simulink library "speedgoatlib"  (Simulink 7.3)
settings: Solver=ode45  StartTime=0.0  StopTime=10.0  RelTol=1e-3
undefined symbols (not defined in the file): m_XR17D15x, mmodemcontrol, standard
libraries: speedgoatlib x176, xpclib x88, simulink x4
(part 1 of 4)
Description:
  | 7.14.0.739 (R2012a)
settings Model: sg_rtwmakecfg_data=_sg_IO75X_v1_2_0_  Creator=dkuratli  LastModifiedBy=lab3
settings Model: ForwardingTableString=|
  | ||__slOldName__||speedgoatlib/Utilities/Disable SMIs||__slNewName__||speedgoatlib_utilities/Disable SMIs||__slOldName__||speedgoatlib/IO101/PMC730 1||__slNewName__||speedgoatlib_IO101/Analog input||__slOldName__||speedgoatlib/IO101/PMC730 2||__slNewName__||speedgoatlib_IO101/Analog output||__slOldName__||speedgoatlib/IO101/PMC730 3||__slNewName__||speedgoatlib_IO101/Digital input||__slOldName__||speedgoatlib/IO101/PMC730 4||__slNewName__||speedgoatlib_IO101/Digital output||__slOldName__||speedgoatlib/IO101/PMC730 5||__slNewName__||speedgoatlib_IO101/Setup||__slOldName__||speedgoatlib/IO102/PMC-16AIO 1||__slNewName__||speedgoatlib_IO102/Setup||__slOldName__||speedgoatlib/IO102/PMC-16AIO 2||__slNewName__||speedgoatlib_IO102/Analog input||__slOldName__||speedgoatlib/IO102/PMC-16AIO 3||__slNewName__||speedgoatlib_IO102/Analog output||__slOldName__||speedgoatlib/IO102/PMC-16AIO 4||__slNewName__||speedgoatlib_IO102/Digital input||__slOldName__||speedgoatlib/IO102/PMC-16AIO 5||__slNewName__||speedgoatlib_IO102/Digital output||__slOldName__||speedgoatlib/IO103/PMC-16AIO168 1||__slNewName__||speedgoatlib_IO103/Setup||__slOldName__||speedgoatlib/IO103/PMC-16AIO168 2||__slNewName__||speedgoatlib_IO103/Analog input||__slOldName__||speedgoatlib/IO103/PMC-16AIO168 3||__slNewName__||speedgoatlib_IO103/Analog output||__slOldName__||speedgoatlib/IO103/PMC-16AIO168 4||__slNewName__||speedgoatlib_IO103/Digital output||__slOldName__||speedgoatlib/IO104/PMC66-16AISS8AO4 1||__slNewName__||speedgoatlib_IO104/Setup||__slOldName__||speedgoatlib/IO104/PMC66-16AISS8AO4 2||__slNewName__||speedgoatlib_IO104/Analog input||__slOldName__||speedgoatlib/IO104/PMC66-16AISS8AO4 3||__slNewName__||speedgoatlib_IO104/Analog output||__slOldName__||speedgoatlib/IO104/PMC66-16AISS8AO4 4||__slNewName__||speedgoatlib_IO104/Digital input||__slOldName__||speedgoatlib/IO104/PMC66-16AISS8AO4 5||__slNewName__||speedgoatlib_IO104/Digital output||__slOldName__||speedgoatlib/IO104/PMC66-16AISS8AO4 6||__slNewName__||speedgoatlib_IO104/Start conversion||__slOldName__||speedgoatlib/IO104/PMC66-16AISS8AO4 7||__slNewName__||speedgoatlib_IO104/Read channels||__slOldName__||speedgoatlib/IO104/PMC66-16AISS8AO4 8||__slNewName__||speedgoatlib_IO104/Update channels||__slOldName__||speedgoatlib/IO104/PMC66-16AISS8AO4 9||__slNewName__||speedgoatlib_IO104/Write channels||__slOldName__||speedgoatlib/IO105/PMC-16AI64 1||__slNewName__||speedgoatlib_IO105/Setup||__slOldName__||speedgoatlib/IO105/PMC-16AI64 2||__slNewName__||speedgoatlib_IO105/Analog input||__slOldName__||speedgoatlib/IO106/PMC66-16AI64SSA 1||__slNewName__||speedgoatlib_IO106/Setup||__slOldName__||speedgoatlib/IO106/PMC66-16AI64SSA 2||__slNewName__||speedgoatlib_IO106/Analog input||__slOldName__||speedgoatlib/IO106/PMC66-16AI64SSA 3||__slNewName__||speedgoatlib_IO106/Start conversion||__slOldName__||speedgoatlib/IO106/PMC66-16AI64SSA 4||__slNewName__||speedgoatlib_IO106/Read channels||__slOldName__||speedgoatlib/IO106/PMC66-16AI64SSA 5||__slNewName__||speedgoatlib_IO106/Analog input (DMA)||__slOldName__||speedgoatlib/IO107/PMC66-16AO16 1||__slNewName__||speedgoatlib_IO107/Setup||__slOldName__||speedgoatlib/IO107/PMC66-16AO16 2||__slNewName__||speedgoatlib_IO107/Analog output||__slOldName__||speedgoatlib/IO108/PMC66-16AO16 1||__slNewName__||speedgoatlib_IO108/Setup||__slOldName__||speedgoatlib/IO108/PMC66-16AO16 2||__slNewName__||speedgoatlib_IO108/Analog output||__slOldName__||speedgoatlib/IO110/TPMC553-10 1||__slNewName__||speedgoatlib_IO110/Setup||__slOldName__||speedgoatlib/IO110/TPMC553-10 2||__slNewName__||speedgoatlib_IO110/Analog output||__slOldName__||speedgoatlib/IO111/TPMC553-11 1||__slNewName__||speedgoatlib_IO111/Setup||__slOldName__||speedgoatlib/IO111/TPMC553-11 2||__slNewName__||speedgoatlib_IO111/Analog output||__slOldName__||speedgoatlib/IO112/PMC66-18AI32SSC 1||__slNewName__||speedgoatlib_IO112/Setup||__slOldName__||speedgoatlib/IO112/PMC66-18AI32SSC 2||__slNewName__||speedgoatlib_IO112/Analog input||__slOldName__||speedgoatlib/IO112/PMC66-18AI32SSC 3||__slNewName__||speedgoatlib_IO112/Start conversion||__slOldName__||speedgoatlib/IO112/PMC66-18AI32SSC 4||__slNewName__||speedgoatlib_IO112/Read channels||__slOldName__||speedgoatlib_io113/Setup||__slNewName__||speedgoatlib_IO113/Setup||__slOldName__||speedgoatlib_io113/Analog output||__slNewName__||speedgoatlib_IO113/Analog output||__slOldName__||speedgoatlib_io113/Digital output||__slNewName__||speedgoatlib_IO113/Digital output||__slOldName__||speedgoatlib_io113/Digital input||__slNewName__||speedgoatlib_IO113/Digital input||__slOldName__||speedgoatlib/IO203/TPMC681 1||__slNewName__||speedgoatlib_IO203/Setup||__slOldName__||speedgoatlib/IO203/TPMC681 2||__slNewName__||speedgoatlib_IO203/Read||__slOldName__||speedgoatlib/IO203/TPMC681 3||__slNewName__||speedgoatlib_IO203/Write||__slOldName__||speedgoatlib/IO204/TPMC671 1||__slNewName__||speedgoatlib_IO204/Setup||__slOldName__||speedgoatlib/IO204/TPMC671 2||__slNewName__||speedgoatlib_IO204/Read||__slOldName__||speedgoatlib/IO204/TPMC671 3||__slNewName__||speedgoatlib_IO204/Write||__slOldName__||speedgoatlib/IO205/TPMC700 1||__slNewName__||speedgoatlib_IO205/Setup||__slOldName__||speedgoatlib/IO205/TPMC700 2||__slNewName__||speedgoatlib_IO205/Read||__slOldName__||speedgoatlib/IO205/TPMC700 3||__slNewName__||speedgoatlib_IO205/Write||__slOldName__||speedgoatlib/IO206/TPMC600 1||__slNewName__||speedgoatlib_IO206/Setup||__slOldName__||speedgoatlib/IO206/TPMC600 2||__slNewName__||speedgoatlib_IO206/Read||__slOldName__||speedgoatlib/IO401/TPMC117 1||__slNewName__||speedgoatlib_IO401/Setup||__slOldName__||speedgoatlib/IO401/TPMC117 2||__slNewName__||speedgoatlib_IO401/Incremental encoder||__slOldName__||speedgoatlib/IO401/TPMC117 3||__slNewName__||speedgoatlib_IO401/Absolute SSI encoder||__slOldName__||speedgoatlib/IO401/TPMC117 4||__slNewName__||speedgoatlib_IO401/Simultaneous read||__slOldName__||speedgoatlib/IO503/TPMC466||__slNewName__||speedgoatlib/IO503/Send Receive||__slOldName__||speedgoatlib/IO503/TEWS TPMC466
  | Internal blocks/Setup ||__slNewName__||speedgoatlib/IO503/Speedgoat IO503
  | Internal blocks/Setup||__slOldName__||speedgoatlib/IO503/TEWS TPMC466
  | Internal blocks/Enable TX ||__slNewName__||speedgoatlib/IO503/Speedgoat IO503
  | Internal blocks/Enable TX||__slOldName__||speedgoatlib/IO503/TEWS TPMC466
  | Internal blocks/Read Int Status||__slNewName__||speedgoatlib/IO503/Speedgoat IO503
  | Internal blocks/Read Int Status||__slOldName__||speedgoatlib/IO503/TEWS TPMC466
  | Internal blocks/Board Setup||__slNewName__||speedgoatlib/IO503/Speedgoat IO503
  | Internal blocks/Board Setup||__slOldName__||speedgoatlib/IO503/TEWS TPMC466
  | Internal blocks/Write HW FIFO||__slNewName__||speedgoatlib/IO503/Speedgoat IO503
  | Internal blocks/Write HW FIFO||__slOldName__||speedgoatlib/IO503/TEWS TPMC466
  | Internal blocks/Read HW FIFO||__slNewName__||speedgoatlib/IO503/Speedgoat IO503
  | Internal blocks/Read HW FIFO||__slOldName__||speedgoatlib/IO503/TEWS TPMC466
  | Internal blocks/Int Source Filter||__slNewName__||speedgoatlib/IO503/Speedgoat IO503
  | Internal blocks/Int Source Filter||__slOldName__||speedgoatlib/IO504/TPMC465||__slNewName__||speedgoatlib/IO504/Send Receive||__slOldName__||speedgoatlib/IO504/TEWS TPMC465
  | Internal blocks/Setup ||__slNewName__||speedgoatlib/IO504/Speedgoat IO504
  | Internal blocks/Setup||__slOldName__||speedgoatlib/IO504/TEWS TPMC465
  | Internal blocks/Read Int Status||__slNewName__||speedgoatlib/IO504/Speedgoat IO504
  | Internal blocks/Read Int Status||__slOldName__||speedgoatlib/IO504/TEWS TPMC465
  | Internal blocks/Board Setup||__slNewName__||speedgoatlib/IO504/Speedgoat IO504
  | Internal blocks/Board Setup||__slOldName__||speedgoatlib/IO504/TEWS TPMC465
  | Internal blocks/Enable TX ||__slNewName__||speedgoatlib/IO504/Speedgoat IO504 Internal blocks/Enable TX||__slOldName__||speedgoatlib/IO504/TEWS TPMC465
  | Internal blocks/Write HW FIFO||__slNewName__||speedgoatlib/IO504/Speedgoat IO504
  | Internal blocks/Write HW FIFO||__slOldName__||speedgoatlib/IO504/TEWS TPMC465
  | Internal blocks/Read HW FIFO||__slNewName__||speedgoatlib/IO504/Speedgoat IO504
  | Internal blocks/Read HW FIFO||__slOldName__||speedgoatlib/IO504/TEWS TPMC465
  | Internal blocks/Int Source Filter||__slNewName__||speedgoatlib/IO504/Speedgoat IO504
  | Internal blocks/Int Source Filter||__slOldName__||speedgoatlib/IO601/iPC-I XC16//PMC 1||__slNewName__||speedgoatlib_IO601/Setup||__slOldName__||speedgoatlib/IO601/iPC-I XC16//PMC 2||__slNewName__||speedgoatlib_IO601/Obsolete/Write||__slOldName__||speedgoatlib/IO601/iPC-I XC16//PMC 3||__slNewName__||speedgoatlib_IO601/Obsolete Read||__slOldName__||speedgoatlib/IO601/iPC-I XC16//PMC 4||__slNewName__||speedgoatlib_IO601/Combined read||__slOldName__||speedgoatlib/IO601/iPC-I XC16//PMC 5||__slNewName__||speedgoatlib_IO601/Status||__slOldName__||speedgoatlib/IO601/iPC-I XC16//PMC 6||__slNewName__||speedgoatlib_IO601/Read status||__slOldName__||speedgoatlib/IO601/iPC-I XC16//PMC 7||__slNewName__||speedgoatlib_IO601/Read status CAN port||__slOldName__||speedgoatlib/IO601/iPC-I XC16//PMC 8||__slNewName__||speedgoatlib_IO601/Send||__slOldName__||speedgoatlib/IO601/iPC-I XC16//PMC 9||__slNewName__||speedgoatlib_IO601/Receive||__slOldName__||speedgoatlib/IO601/iPC-I XC16//PMC 12 v2||__slNewName__||speedgoatlib_IO601/Write||__slOldName__||speedgoatlib/IO601/iPC-I XC16//PMC 13 v2||__slNewName__||speedgoatlib_IO601/Read

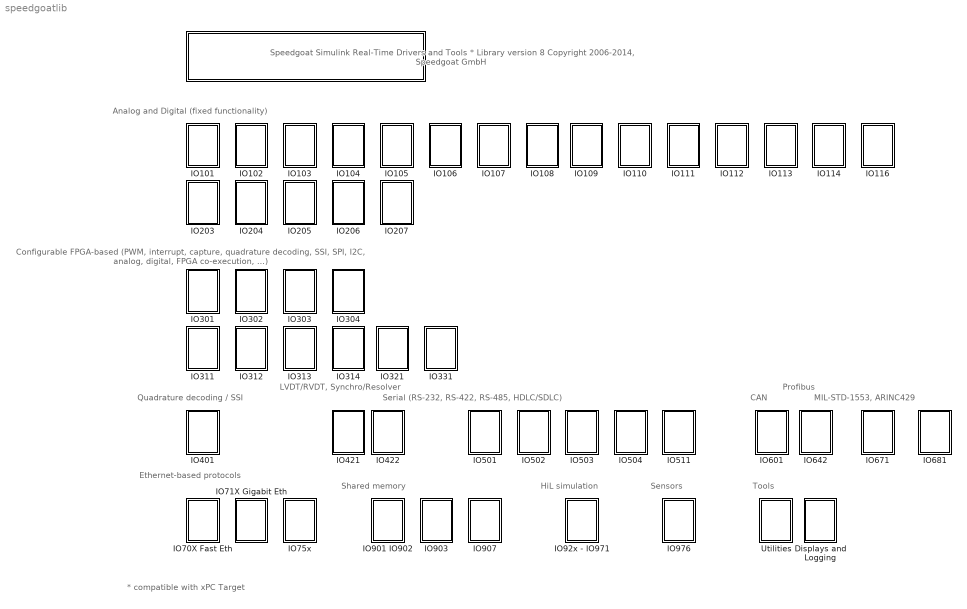
== system speedgoatlib ==
  note: * compatible with xPC Target
  note: Speedgoat Simulink Real-Time Drivers and Tools *
      | Library version 8
      | Copyright 2006-2014, Speedgoat GmbH
  note: Analog and Digital (fixed functionality)
  note: Configurable FPGA-based (PWM, interrupt, capture, quadrature decoding, SSI, SPI, I2C, analog, digital, FPGA co-execution, ...)
  note: Quadrature decoding / SSI
  note: Serial (RS-232, RS-422, RS-485, HDLC/SDLC)
  note: CAN
  note: Ethernet-based protocols
  note: Shared memory
  note: Tools
  note: HiL simulation
  note: Sensors
  note: MIL-STD-1553, ARINC429
  note: LVDT/RVDT, Synchro/Resolver
  note: Profibus
  " " : Subsystem
      settings: OpenFcn=;
      mask Display: image(imread('sg_logo.png'))
  Displays and Logging : Subsystem
      settings: OpenFcn=|
      | [matlabVer, count] = sscanf(version, '%i.%i.%i');
      | 
      | if (matlabVer(1) < 7) || ( (matlabVer(1) == 8) && (matlabVer(2) <= 2) )
      |   load_system('xpclib');
      |   open_system('xpclib/Misc.');
      | else
      |   load_system('slrtlib');
      |   open_system('slrtlib/Displays and Logging');
      | end
  IO101 : Subsystem
      settings: OpenFcn=speedgoatlib_IO101
  IO102 : Subsystem
      settings: OpenFcn=speedgoatlib_IO102
  IO103 : Subsystem
      settings: OpenFcn=speedgoatlib_IO103
  IO104 : Subsystem
      settings: OpenFcn=speedgoatlib_IO104
  IO105 : Subsystem
      settings: OpenFcn=speedgoatlib_IO105
  IO106 : Subsystem
      settings: OpenFcn=speedgoatlib_IO106
  IO107 : Subsystem
      settings: OpenFcn=speedgoatlib_IO107
  IO108 : Subsystem
      settings: OpenFcn=speedgoatlib_IO108
  IO109 : Subsystem
      settings: OpenFcn=speedgoatlib_IO109
  IO110 : Subsystem
      settings: OpenFcn=speedgoatlib_IO110
  IO111 : Subsystem
      settings: OpenFcn=speedgoatlib_IO111
  IO112 : Subsystem
      settings: OpenFcn=speedgoatlib_IO112
  IO113 : Subsystem
      settings: OpenFcn=speedgoatlib_IO113
  IO114 : Subsystem
      settings: OpenFcn=speedgoatlib_IO114
  IO116 : Subsystem
      settings: OpenFcn=speedgoatlib_IO116
  IO203 : Subsystem
      settings: OpenFcn=speedgoatlib_IO203
  IO204 : Subsystem
      settings: OpenFcn=speedgoatlib_IO204
  IO205 : Subsystem
      settings: OpenFcn=speedgoatlib_IO205
  IO206 : Subsystem
      settings: OpenFcn=speedgoatlib_IO206
  IO207 : Subsystem
      settings: OpenFcn=speedgoatlib_IO207
  IO301 : Subsystem
      settings: OpenFcn=speedgoatlib_IO301
  IO302 : Subsystem
      settings: OpenFcn=speedgoatlib_IO302
  IO303 : Subsystem
      settings: OpenFcn=speedgoatlib_IO303
  IO304 : Subsystem
      settings: OpenFcn=speedgoatlib_IO304
  IO311 : Subsystem
      settings: OpenFcn=speedgoatlib_IO311
  IO312 : Subsystem
      settings: OpenFcn=speedgoatlib_IO312
  IO313 : Subsystem
      settings: OpenFcn=speedgoatlib_IO313
  IO314 : Subsystem
      settings: OpenFcn=speedgoatlib_IO314
  IO321 : Subsystem
      settings: OpenFcn=speedgoatlib_IO321
  IO331 : Subsystem
      settings: OpenFcn=speedgoatlib_fpga
  IO401 : Subsystem
      settings: OpenFcn=speedgoatlib_IO401
  IO421 : Subsystem
      settings: OpenFcn=speedgoatlib_IO421
  IO422 : Subsystem
      settings: OpenFcn=speedgoatlib_IO422
  IO501 : Subsystem
  IO502 : Subsystem
  IO503 : Subsystem
  IO504 : Subsystem
  IO511 : Subsystem
      settings: OpenFcn=speedgoatlib_IO511
  IO601 : Subsystem
      settings: OpenFcn=speedgoatlib_IO601
  IO642 : Subsystem
      settings: OpenFcn=speedgoatlib_IO642
  IO671 : Subsystem
      settings: OpenFcn=|
      | load_system('xpccondorlib');
      | open_system('xpccondorlib/MIL-STD 1553');
  IO681 : Subsystem
      settings: OpenFcn=|
      | load_system('xpccondorlib');
      | open_system('xpccondorlib/ARINC-429');
  IO70X Fast Eth : Subsystem
      settings: OpenFcn=speedgoatlib_IO70X
  IO71X Gigabit Eth : Subsystem
      settings: OpenFcn=speedgoatlib_IO71X
  IO75x : Subsystem
      settings: OpenFcn=speedgoatlib_IO75X
  IO901 IO902 : Subsystem
      settings: OpenFcn=cwcec_scgtLib
  IO903 : Subsystem
      settings: OpenFcn=|
      | open_system('xpcsystranlib');
      | open_system('xpcsystranlib/Shared Memory');
  IO907 : Subsystem
      settings: OpenFcn=|
      | load_system('xpcgefanuclib');
      | open_system('xpcgefanuclib/Shared Memory');
  IO92x - IO971 : Subsystem
      settings: OpenFcn=speedgoatlib_PIL
  IO976 : Subsystem
      settings: OpenFcn=|
      | load_system('xpcmeasurementcomputinglib');
      | open_system('xpcmeasurementcomputinglib/Thermo couple');
  Utilities : Subsystem
      settings: OpenFcn=speedgoatlib_utilities

== system speedgoatlib/  ==

== system speedgoatlib/Displays and Logging ==

== system speedgoatlib/IO101 ==

== system speedgoatlib/IO102 ==

== system speedgoatlib/IO103 ==

== system speedgoatlib/IO104 ==

== system speedgoatlib/IO105 ==

== system speedgoatlib/IO106 ==

== system speedgoatlib/IO107 ==

== system speedgoatlib/IO108 ==

== system speedgoatlib/IO109 ==

== system speedgoatlib/IO110 ==

== system speedgoatlib/IO111 ==

== system speedgoatlib/IO112 ==

== system speedgoatlib/IO113 ==

== system speedgoatlib/IO114 ==

== system speedgoatlib/IO116 ==

== system speedgoatlib/IO203 ==

== system speedgoatlib/IO204 ==

== system speedgoatlib/IO205 ==

== system speedgoatlib/IO206 ==

== system speedgoatlib/IO207 ==

== system speedgoatlib/IO301 ==

== system speedgoatlib/IO302 ==

== system speedgoatlib/IO303 ==

== system speedgoatlib/IO304 ==

== system speedgoatlib/IO311 ==

== system speedgoatlib/IO312 ==

== system speedgoatlib/IO313 ==

== system speedgoatlib/IO314 ==

== system speedgoatlib/IO321 ==

== system speedgoatlib/IO331 ==

== system speedgoatlib/IO401 ==

== system speedgoatlib/IO421 ==

== system speedgoatlib/IO422 ==

== system speedgoatlib/IO501 ==
  Acromag PMC520 Internal blocks : Subsystem
  Modem Control : S-Function  InitFcn=mmodemcontrol(3)  FunctionName=modem_control_XR17D15x  Parameters=slot, port, boardtype, rts, dtr, count  EnableBusSupport=off  mask(modem_control_XR17D15x){port=1, rts=on, dtr=off, slot=[2,13]}
      mask prompts: slot "PCI slot: (-1 for autosearch)"
      mask help:
      | PMC520
      | Acromag
      | Modem Control
      mask init:
      | count = 0;
      | boardtype = 100;
      | [maskdisplay, count] = mmodemcontrol( 2, rts, dtr, boardtype, 0, 0 );
      | set_param( gcb, 'MaskDisplay', maskdisplay );
      mask Help: helpview(fullfile(docroot, 'mapfiles', 'xpc.map'), 'Quatech_MODEM_Control')
      mask StyleString: popup(1|2),checkbox,checkbox,edit
      mask Display: disp('PMC520\nAcromag\nModem Control');port_label('input',1,'RTS');
  Modem Status : S-Function  FunctionName=modem_status_XR17D15x  Parameters=slot, port, boardtype, cts, dsr, ring, dcd, count, sampletime  EnableBusSupport=off  mask(modem_status_XR17D15x){port=1, cts=on, dsr=off, ring=off, dcd=off, sampletime=-1, slot=[2,13]}
      mask prompts: ring "RI:"; slot "PCI slot: (-1 for autosearch)"
      mask help:
      | PMC520
      | Acromag
      | Modem Status
      mask init:
      | count = 0;
      | boardtype = 100;
      | [maskdisplay, count] = mmodemstatus( 2, cts, dsr, ring, dcd, boardtype );
      | set_param( gcb, 'MaskDisplay', maskdisplay );
      mask Help: helpview(fullfile(docroot, 'mapfiles', 'xpc.map'), 'FC422_MODEM_Status')
      mask StyleString: popup(1|2),checkbox,checkbox,checkbox,checkbox,edit,edit
      mask Display: disp('PMC520\nAcromag\nModem Control');port_label('output',1,'CTS');
  PMC520 : Subsystem  InitFcn=m_XR17D15x(3);  mask(RS232 Send Receive){group=Board Setup, port=1, irqnum=5, clockfreq=14745600, standard=on, slot=-1, baud1=115200, bauddivisor1=1, sampling1=16x (standard), prescale1=off, parity1=None, ndata1=8, nstop1=1, rlevel1=1, hwmode1=none, swmode1=none, xonchar1=17, xoffchar1=19, rs485auto1=off, rs485delay1=0, xmtfifosize1=1024, xmtdatatype1=8 bit uint null terminated, rcvfifosize1=1024, baud2=115200, bauddivisor2=1, sampling2=16x (standard), prescale2=off, parity2=None, ndata2=8, nstop2=1, rlevel2=1, hwmode2=none, swmode2=none, xonchar2=17, xoffchar2=19, rs485auto2=off, rs485delay2=0, xmtfifosize2=1024, xmtdatatype2=8 bit uint null terminated, rcvfifosize2=1024, baud3=115200, bauddivisor3=1, sampling3=16x (standard), prescale3=off, parity3=None, ndata3=8, nstop3=1, rlevel3=half full (32), hwmode3=none, swmode3=none, xonchar3=17, xoffchar3=19, rs485auto3=off, rs485delay3=0, xmtfifosize3=1024, xmtdatatype3=8 bit uint null terminated, rcvfifosize3=1024, baud4=115200, bauddivisor4=1, sampling4=16x (standard), prescale4=off, parity4=None, ndata4=8, nstop4=1, rlevel4=half full (32), hwmode4=none, swmode4=none, xonchar4=17, xoffchar4=19, rs485auto4=off, rs485delay4=0, xmtfifosize4=1024, xmtdatatype4=8 bit uint null terminated, rcvfifosize4=1024, baud5=115200, bauddivisor5=1, sampling5=16x (standard), prescale5=off, parity5=None, ndata5=8, nstop5=1, rlevel5=1, hwmode5=none, swmode5=none, xonchar5=17, xoffchar5=19, rs485auto5=off, rs485delay5=0, xmtfifosize5=1024, xmtdatatype5=8 bit uint null terminated, rcvfifosize5=1024, baud6=115200, bauddivisor6=1, sampling6=16x (standard), prescale6=off, parity6=None, ndata6=8, nstop6=1, rlevel6=1, hwmode6=none, swmode6=none, xonchar6=17, xoffchar6=19, rs485auto6=off, rs485delay6=0, xmtfifosize6=1024, xmtdatatype6=8 bit uint null terminated, rcvfifosize6=1024, baud7=115200, bauddivisor7=1, sampling7=16x (standard), prescale7=off, parity7=None, ndata7=8, nstop7=1, rlevel7=1, hwmode7=none, swmode7=none, xonchar7=17, xoffchar7=19, rs485auto7=off, rs485delay7=0, xmtfifosize7=1024, xmtdatatype7=8 bit uint null terminated, rcvfifosize7=1024, baud8=115200, bauddivisor8=1, sampling8=16x (standard), prescale8=off, parity8=None, ndata8=8, nstop8=1, rlevel8=1, hwmode8=none, swmode8=none, xonchar8=17, xoffchar8=19, rs485auto8=off, rs485delay8=0, xmtfifosize8=1024, xmtdatatype8=8 bit uint null terminated, rcvfifosize8=1024}
      mask prompts: group "Parameter group:"; port "Port to modify:"; irqnum "IRQ number:"; clockfreq "Master Clock Frequeny (standard = 14.7456E6 Hz):"; standard "Use standard reference and rates (Ref = 14.7456E6 Hz, 16x sampling, all ports)"; baud1 "Baud rate:"; bauddivisor1 "Baud divisor:"; sampling1 "Sampling rate:"; prescale1 "Prescale (divide reference by 4)"; parity1 "Parity:"; ndata1 "Data bits:"; nstop1 "Stop bits:"; rlevel1 "Receive FIFO interrupt level:"; hwmode1 "Hardware handshake:"; swmode1 "Software handshake:"; xonchar1 "XON character:"; xoffchar1 "XOFF character:"; rs485auto1 "RS485 auto turnaround:"; rs485delay1 "RS485 turnaround delay [0,15]"; xmtfifosize1 "Transmit software FIFO size:"; xmtdatatype1 "Transmit FIFO data type:"; rcvfifosize1 "Receive software FIFO size:"; baud2 "Baud rate:"; bauddivisor2 "Baud divisor:"; sampling2 "Sampling rate:"; prescale2 "Prescale (divide reference by 4)"; parity2 "Parity:"; ndata2 "Data bits:"; nstop2 "Stop bits:"; rlevel2 "Receive FIFO interrupt level:"; hwmode2 "Hardware handshake:"; swmode2 "Software handshake:"; xonchar2 "XON character:"; xoffchar2 "XOFF character:"; rs485auto2 "RS485 auto turnaround:"; rs485delay2 "RS485 turnaround delay [0,15]"; xmtfifosize2 "Transmit software FIFO size:"; xmtdatatype2 "Transmit FIFO data type:"; rcvfifosize2 "Receive software FIFO size:"; baud3 "Baud rate:"; bauddivisor3 "Baud divisor:"; sampling3 "Sampling rate:"; prescale3 "Prescale (divide reference by 4)"; parity3 "Parity:"; ndata3 "Data bits:"; nstop3 "Stop bits:"; rlevel3 "Receive FIFO interrupt level:"; hwmode3 "Hardware handshake:"; swmode3 "Software handshake:"; xonchar3 "XON character:"; xoffchar3 "XOFF character:"; rs485auto3 "RS485 auto turnaround:"; rs485delay3 "RS485 turnaround delay [0,15]"; xmtfifosize3 "Transmit software FIFO size:"; xmtdatatype3 "Transmit FIFO data type:"; rcvfifosize3 "Receive software FIFO size:"; baud4 "Baud rate:"; bauddivisor4 "Baud divisor:"; sampling4 "Sampling rate:"; prescale4 "Prescale (divide reference by 4)"; parity4 "Parity:"; ndata4 "Data bits:"; nstop4 "Stop bits:"; rlevel4 "Receive FIFO interrupt level:"; hwmode4 "Hardware handshake:"; swmode4 "Software handshake:"; xonchar4 "XON character:"; xoffchar4 "XOFF character:"; rs485auto4 "RS485 auto turnaround:"; rs485delay4 "RS485 turnaround delay [0,15]"; xmtfifosize4 "Transmit software FIFO size:"; xmtdatatype4 "Transmit FIFO data type:"; rcvfifosize4 "Receive software FIFO size:"; baud5 "Baud rate:"; bauddivisor5 "Baud divisor:"; sampling5 "Sampling rate:"; prescale5 "Prescale (divide reference by 4)"; parity5 "Parity:"; ndata5 "Data bits:"; nstop5 "Stop bits:"; rlevel5 "Receive FIFO interrupt level:"; hwmode5 "Hardware handshake:"; swmode5 "Software handshake:"; xonchar5 "XON character:"; xoffchar5 "XOFF character:"; rs485auto5 "RS485 auto turnaround:"; rs485delay5 "RS485 turnaround delay [0,15]"; xmtfifosize5 "Transmit software FIFO size:"; xmtdatatype5 "Transmit FIFO data type:"; rcvfifosize5 "Receive software FIFO size:"; baud6 "Baud rate:"; bauddivisor6 "Baud divisor:"; sampling6 "Sampling rate:"; prescale6 "Prescale (divide reference by 4)"; parity6 "Parity:"; ndata6 "Data bits:"; nstop6 "Stop bits:"; rlevel6 "Receive FIFO interrupt level:"; hwmode6 "Hardware handshake:"; swmode6 "Software handshake:"; xonchar6 "XON character:"; xoffchar6 "XOFF character:"; rs485auto6 "RS485 auto turnaround:"; rs485delay6 "RS485 turnaround delay [0,15]"; xmtfifosize6 "Transmit software FIFO size:"; xmtdatatype6 "Transmit FIFO data type:"; rcvfifosize6 "Receive software FIFO size:"; baud7 "Baud rate:"; bauddivisor7 "Baud divisor:"; sampling7 "Sampling rate:"; prescale7 "Prescale (divide reference by 4)"; parity7 "Parity:"; ndata7 "Data bits:"; nstop7 "Stop bits:"; rlevel7 "Receive FIFO interrupt level:"; hwmode7 "Hardware handshake:"; swmode7 "Software handshake:"; xonchar7 "XON character:"; xoffchar7 "XOFF character:"; rs485auto7 "RS485 auto turnaround:"; rs485delay7 "RS485 turnaround delay [0,15]"; xmtfifosize7 "Transmit software FIFO size:"; xmtdatatype7 "Transmit FIFO data type:"; rcvfifosize7 "Receive software FIFO size:"; baud8 "Baud rate:"; bauddivisor8 "Baud divisor:"; sampling8 "Sampling rate:"; prescale8 "Prescale (divide reference by 4)"; parity8 "Parity:"; ndata8 "Data bits:"; nstop8 "Stop bits:"; rlevel8 "Receive FIFO interrupt level:"; hwmode8 "Hardware handshake:"; swmode8 "Software handshake:"; xonchar8 "XON character:"; xoffchar8 "XOFF character:"; rs485auto8 "RS485 auto turnaround:"; rs485delay8 "RS485 turnaround delay [0,15]"; xmtfifosize8 "Transmit software FIFO size:"; xmtdatatype8 "Transmit FIFO data type:"; rcvfifosize8 "Receive software FIFO size:"
      mask help:
      | PMC520
      | Acromag
      | RS232 Send Receive Subsystem
      mask init:
      | brdslot = slot;
      | m_XR17D15x(1, 8);
      mask Help: helpview(fullfile(docroot, 'mapfiles', 'xpc.map'), 'Commtech_Subsystem')
      mask StyleString: popup(Board Setup|Basic Setup|FIFO Setup),popup(1|2|3|4|5|6|7|8),edit,edit,checkbox,edit,popup(921600|460800|230400|115200|57600|38400|19200|9600|4800|2400|1200|600|300|110),edit,popup(8x|16x (standard)),checkbox,popup(None|Even|Odd|Mark|Space),popup(5|6|7|8),popup(1|2),popup(1|quarter full (16)|half full (32)|almost full (56)),popup(RTS/CTS|none),popup(XON/XOFF|none),edit,edit,checkbox,edit,edit,popup(count+32 bit int|count+32 bit uint|count+16 bit int|count+16 bit uint|8 bit int null terminated|8 bit uint null terminated),edit,popup(921600|460800|230400|115200|57600|38400|19200|9600|4800|2400|1200|600|300|110),edit,popup(8x|16x (standard)),checkbox,popup(None|Even|Odd|Mark|Space),popup(5|6|7|8),popup(1|2),popup(1|quarter full (16)|half full (32)|almost full (56)),popup(RTS/CTS|none),popup(XON/XOFF|none),edit,edit,checkbox,edit,edit,popup(count+32 bit int|count+32 bit uint|count+16 bit int|count+16 bit uint|8 bit int null terminated|8 bit uint null terminated),edit,popup(921600|460800|230400|115200|57600|38400|19200|9600|4800|2400|1200|600|300|110),edit,popup(8x|16x (standard)),checkbox,popup(None|Even|Odd|Mark|Space),popup(5|6|7|8),popup(1|2),popup(1|quarter full (16)|half full (32)|almost full (56)),popup(RTS/CTS|none),popup(XON/XOFF|none),edit,edit,checkbox,edit,edit,popup(count+32 bit int|count+32 bit uint|count+16 bit int|count+16 bit uint|8 bit int null terminated|8 bit uint null terminated),edit,popup(921600|460800|230400|115200|57600|38400|19200|9600|4800|2400|1200|600|300|110),edit,popup(8x|16x (standard)),checkbox,popup(None|Even|Odd|Mark|Space),popup(5|6|7|8),popup(1|2),popup(1|quarter full (16)|half full (32)|almost full (56)),popup(RTS/CTS|none),popup(XON/XOFF|none),edit,edit,checkbox,edit,edit,popup(count+32 bit int|count+32 bit uint|count+16 bit int|count+16 bit uint|8 bit int null terminated|8 bit uint null terminated),edit,popup(921600|460800|230400|115200|57600|38400|19200|9600|4800|2400|1200|600|300|110),edit,popup(8x|16x (standard)),checkbox,popup(None|Even|Odd|Mark|Space),popup(5|6|7|8),popup(1|2),popup(1|quarter full (16)|half full (32)|almost full (56)),popup(RTS/CTS|none),popup(XON/XOFF|none),edit,edit,checkbox,edit,edit,popup(count+32 bit int|count+32 bit uint|count+16 bit int|count+16 bit uint|8 bit int null terminated|8 bit uint null terminated),edit,popup(921600|460800|230400|115200|57600|38400|19200|9600|4800|2400|1200|600|300|110),edit,popup(8x|16x (standard)),checkbox,popup(None|Even|Odd|Mark|Space),popup(5|6|7|8),popup(1|2),popup(1|quarter full (16)|half full (32)|almost full (56)),popup(RTS/CTS|none),popup(XON/XOFF|none),edit,edit,checkbox,edit,edit,popup(count+32 bit int|count+32 bit uint|count+16 bit int|count+16 bit uint|8 bit int null terminated|8 bit uint null terminated),edit,popup(921600|460800|230400|115200|57600|38400|19200|9600|4800|2400|1200|600|300|110),edit,popup(8x|16x (standard)),checkbox,popup(None|Even|Odd|Mark|Space),popup(5|6|7|8),popup(1|2),popup(1|quarter full (16)|half full (32)|almost full (56)),popup(RTS/CTS|none),popup(XON/XOFF|none),edit,edit,checkbox,edit,edit,popup(count+32 bit int|count+32 bit uint|count+16 bit int|count+16 bit uint|8 bit int null terminated|8 bit uint null terminated),edit,popup(921600|460800|230400|115200|57600|38400|19200|9600|4800|2400|1200|600|300|110),edit,popup(8x|16x (standard)),checkbox,popup(None|Even|Odd|Mark|Space),popup(5|6|7|8),popup(1|2),popup(1|quarter full (16)|half full (32)|almost full (56)),popup(RTS/CTS|none),popup(XON/XOFF|none),edit,edit,checkbox,edit,edit,popup(count+32 bit int|count+32 bit uint|count+16 bit int|count+16 bit uint|8 bit int null terminated|8 bit uint null terminated),edit
      mask CallbackString:
      | m_XR17D15x(2, 8);|m_XR17D15x(2, 8);|||m_XR17D15x(2, 8);
      | |||||||||||||||||||||||||||||||||||||||||||||||||||||||||||||||||||||||||||||||||||||||||||||||||||||||||||||||||||||||||||||||||||||||||
      mask Display:
      | disp('Acromag\nPMC520\nRS-232\nSend\nReceive');
      | port_label( 'input', 1, 'XMT1' );
      | port_label( 'input', 2, 'XMT2' );
      | port_label( 'input', 3, 'XMT3' );
      | port_label( 'input', 4, 'XMT4' );
      | port_label( 'input', 5, 'XMT5' );
      | port_label( 'input', 6, 'XMT6' );
      | port_label( 'input', 7, 'XMT7' );
      | port_label( 'input', 8, 'XMT8' );
      | 
      | port_label( 'output', 1, 'FIFO1' );
      | port_label( 'output', 2, 'FIFO2' );
      | port_label( 'output', 3, 'FIFO3' );
      | port_label( 'output', 4, 'FIFO4' );
      | port_label( 'output', 5, 'FIFO5' );
      | port_label( 'output', 6, 'FIFO6' );
      | port_label( 'output', 7, 'FIFO7' );
      | port_label( 'output', 8, 'FIFO8' );

== system speedgoatlib/IO502 ==
  Acromag PMC521 Internal blocks : Subsystem
  Modem Control : S-Function  InitFcn=mmodemcontrol(3)  FunctionName=modem_control_XR17D15x  Parameters=slot, port, boardtype, rts, dtr, count  EnableBusSupport=off  mask(modem_control_XR17D15x){port=1, rts=on, dtr=off, slot=[2,13]}
      mask prompts: slot "PCI slot: (-1 for autosearch)"
      mask help:
      | PMC521
      | Acromag
      | Modem Control
      mask init:
      | count = 0;
      | boardtype = 101;
      | [maskdisplay, count] = mmodemcontrol( 2, rts, dtr, boardtype, 0, 0 );
      | set_param( gcb, 'MaskDisplay', maskdisplay );
      mask Help: helpview(fullfile(docroot, 'mapfiles', 'xpc.map'), 'Quatech_MODEM_Control')
      mask StyleString: popup(1|2),checkbox,checkbox,edit
      mask Display: disp('Speedgoat\nIO502\nModem Control');port_label('input',1,'RTS');
  Modem Status : S-Function  FunctionName=modem_status_XR17D15x  Parameters=slot, port, boardtype, cts, dsr, ring, dcd, count, sampletime  EnableBusSupport=off  mask(modem_status_XR17D15x){port=1, cts=on, dsr=off, ring=off, dcd=off, sampletime=-1, slot=[2,13]}
      mask prompts: ring "RI:"; slot "PCI slot: (-1 for autosearch)"
      mask help:
      | PMC521
      | Acromag
      | Modem Status
      mask init:
      | count = 0;
      | boardtype = 101;
      | [maskdisplay, count] = mmodemstatus( 2, cts, dsr, ring, dcd, boardtype );
      | set_param( gcb, 'MaskDisplay', maskdisplay );
      mask Help: helpview(fullfile(docroot, 'mapfiles', 'xpc.map'), 'FC422_MODEM_Status')
      mask StyleString: popup(1|2),checkbox,checkbox,checkbox,checkbox,edit,edit
      mask Display: disp('Speedgoat\nIO502\nModem Status');port_label('output',1,'CTS');
  PMC521 : Subsystem  InitFcn=m_XR17D15x(3);  mask(RS232 Send Receive){group=Board Setup, port=1, irqnum=5, clockfreq=14745600, standard=on, slot=-1, baud1=115200, bauddivisor1=1, sampling1=16x (standard), prescale1=off, parity1=None, ndata1=8, nstop1=1, rlevel1=1, hwmode1=none, swmode1=none, xonchar1=17, xoffchar1=19, rs485auto1=off, rs485delay1=0, xmtfifosize1=1024, xmtdatatype1=8 bit uint null terminated, rcvfifosize1=1024, baud2=115200, bauddivisor2=1, sampling2=16x (standard), prescale2=off, parity2=None, ndata2=8, nstop2=1, rlevel2=1, hwmode2=none, swmode2=none, xonchar2=17, xoffchar2=19, rs485auto2=off, rs485delay2=0, xmtfifosize2=1024, xmtdatatype2=8 bit uint null terminated, rcvfifosize2=1024, baud3=115200, bauddivisor3=1, sampling3=16x (standard), prescale3=off, parity3=None, ndata3=8, nstop3=1, rlevel3=half full (32), hwmode3=none, swmode3=none, xonchar3=17, xoffchar3=19, rs485auto3=off, rs485delay3=0, xmtfifosize3=1024, xmtdatatype3=8 bit uint null terminated, rcvfifosize3=1024, baud4=115200, bauddivisor4=1, sampling4=16x (standard), prescale4=off, parity4=None, ndata4=8, nstop4=1, rlevel4=half full (32), hwmode4=none, swmode4=none, xonchar4=17, xoffchar4=19, rs485auto4=off, rs485delay4=0, xmtfifosize4=1024, xmtdatatype4=8 bit uint null terminated, rcvfifosize4=1024, baud5=115200, bauddivisor5=1, sampling5=16x (standard), prescale5=off, parity5=None, ndata5=8, nstop5=1, rlevel5=1, hwmode5=none, swmode5=none, xonchar5=17, xoffchar5=19, rs485auto5=off, rs485delay5=0, xmtfifosize5=1024, xmtdatatype5=8 bit uint null terminated, rcvfifosize5=1024, baud6=115200, bauddivisor6=1, sampling6=16x (standard), prescale6=off, parity6=None, ndata6=8, nstop6=1, rlevel6=1, hwmode6=none, swmode6=none, xonchar6=17, xoffchar6=19, rs485auto6=off, rs485delay6=0, xmtfifosize6=1024, xmtdatatype6=8 bit uint null terminated, rcvfifosize6=1024, baud7=115200, bauddivisor7=1, sampling7=16x (standard), prescale7=off, parity7=None, ndata7=8, nstop7=1, rlevel7=1, hwmode7=none, swmode7=none, xonchar7=17, xoffchar7=19, rs485auto7=off, rs485delay7=0, xmtfifosize7=1024, xmtdatatype7=8 bit uint null terminated, rcvfifosize7=1024, baud8=115200, bauddivisor8=1, sampling8=16x (standard), prescale8=off, parity8=None, ndata8=8, nstop8=1, rlevel8=1, hwmode8=none, swmode8=none, xonchar8=17, xoffchar8=19, rs485auto8=off, rs485delay8=0, xmtfifosize8=1024, xmtdatatype8=8 bit uint null terminated, rcvfifosize8=1024}
      mask prompts: group "Parameter group:"; port "Port to modify:"; irqnum "IRQ number:"; clockfreq "Master Clock Frequeny (standard = 14.7456E6 Hz):"; standard "Use standard reference and rates (Ref = 14.7456E6 Hz, 16x sampling, all ports)"; baud1 "Baud rate:"; bauddivisor1 "Baud divisor:"; sampling1 "Sampling rate:"; prescale1 "Prescale (divide reference by 4)"; parity1 "Parity:"; ndata1 "Data bits:"; nstop1 "Stop bits:"; rlevel1 "Receive FIFO interrupt level:"; hwmode1 "Hardware handshake:"; swmode1 "Software handshake:"; xonchar1 "XON character:"; xoffchar1 "XOFF character:"; rs485auto1 "RS485 auto turnaround:"; rs485delay1 "RS485 turnaround delay [0,15]"; xmtfifosize1 "Transmit software FIFO size:"; xmtdatatype1 "Transmit FIFO data type:"; rcvfifosize1 "Receive software FIFO size:"; baud2 "Baud rate:"; bauddivisor2 "Baud divisor:"; sampling2 "Sampling rate:"; prescale2 "Prescale (divide reference by 4)"; parity2 "Parity:"; ndata2 "Data bits:"; nstop2 "Stop bits:"; rlevel2 "Receive FIFO interrupt level:"; hwmode2 "Hardware handshake:"; swmode2 "Software handshake:"; xonchar2 "XON character:"; xoffchar2 "XOFF character:"; rs485auto2 "RS485 auto turnaround:"; rs485delay2 "RS485 turnaround delay [0,15]"; xmtfifosize2 "Transmit software FIFO size:"; xmtdatatype2 "Transmit FIFO data type:"; rcvfifosize2 "Receive software FIFO size:"; baud3 "Baud rate:"; bauddivisor3 "Baud divisor:"; sampling3 "Sampling rate:"; prescale3 "Prescale (divide reference by 4)"; parity3 "Parity:"; ndata3 "Data bits:"; nstop3 "Stop bits:"; rlevel3 "Receive FIFO interrupt level:"; hwmode3 "Hardware handshake:"; swmode3 "Software handshake:"; xonchar3 "XON character:"; xoffchar3 "XOFF character:"; rs485auto3 "RS485 auto turnaround:"; rs485delay3 "RS485 turnaround delay [0,15]"; xmtfifosize3 "Transmit software FIFO size:"; xmtdatatype3 "Transmit FIFO data type:"; rcvfifosize3 "Receive software FIFO size:"; baud4 "Baud rate:"; bauddivisor4 "Baud divisor:"; sampling4 "Sampling rate:"; prescale4 "Prescale (divide reference by 4)"; parity4 "Parity:"; ndata4 "Data bits:"; nstop4 "Stop bits:"; rlevel4 "Receive FIFO interrupt level:"; hwmode4 "Hardware handshake:"; swmode4 "Software handshake:"; xonchar4 "XON character:"; xoffchar4 "XOFF character:"; rs485auto4 "RS485 auto turnaround:"; rs485delay4 "RS485 turnaround delay [0,15]"; xmtfifosize4 "Transmit software FIFO size:"; xmtdatatype4 "Transmit FIFO data type:"; rcvfifosize4 "Receive software FIFO size:"; baud5 "Baud rate:"; bauddivisor5 "Baud divisor:"; sampling5 "Sampling rate:"; prescale5 "Prescale (divide reference by 4)"; parity5 "Parity:"; ndata5 "Data bits:"; nstop5 "Stop bits:"; rlevel5 "Receive FIFO interrupt level:"; hwmode5 "Hardware handshake:"; swmode5 "Software handshake:"; xonchar5 "XON character:"; xoffchar5 "XOFF character:"; rs485auto5 "RS485 auto turnaround:"; rs485delay5 "RS485 turnaround delay [0,15]"; xmtfifosize5 "Transmit software FIFO size:"; xmtdatatype5 "Transmit FIFO data type:"; rcvfifosize5 "Receive software FIFO size:"; baud6 "Baud rate:"; bauddivisor6 "Baud divisor:"; sampling6 "Sampling rate:"; prescale6 "Prescale (divide reference by 4)"; parity6 "Parity:"; ndata6 "Data bits:"; nstop6 "Stop bits:"; rlevel6 "Receive FIFO interrupt level:"; hwmode6 "Hardware handshake:"; swmode6 "Software handshake:"; xonchar6 "XON character:"; xoffchar6 "XOFF character:"; rs485auto6 "RS485 auto turnaround:"; rs485delay6 "RS485 turnaround delay [0,15]"; xmtfifosize6 "Transmit software FIFO size:"; xmtdatatype6 "Transmit FIFO data type:"; rcvfifosize6 "Receive software FIFO size:"; baud7 "Baud rate:"; bauddivisor7 "Baud divisor:"; sampling7 "Sampling rate:"; prescale7 "Prescale (divide reference by 4)"; parity7 "Parity:"; ndata7 "Data bits:"; nstop7 "Stop bits:"; rlevel7 "Receive FIFO interrupt level:"; hwmode7 "Hardware handshake:"; swmode7 "Software handshake:"; xonchar7 "XON character:"; xoffchar7 "XOFF character:"; rs485auto7 "RS485 auto turnaround:"; rs485delay7 "RS485 turnaround delay [0,15]"; xmtfifosize7 "Transmit software FIFO size:"; xmtdatatype7 "Transmit FIFO data type:"; rcvfifosize7 "Receive software FIFO size:"; baud8 "Baud rate:"; bauddivisor8 "Baud divisor:"; sampling8 "Sampling rate:"; prescale8 "Prescale (divide reference by 4)"; parity8 "Parity:"; ndata8 "Data bits:"; nstop8 "Stop bits:"; rlevel8 "Receive FIFO interrupt level:"; hwmode8 "Hardware handshake:"; swmode8 "Software handshake:"; xonchar8 "XON character:"; xoffchar8 "XOFF character:"; rs485auto8 "RS485 auto turnaround:"; rs485delay8 "RS485 turnaround delay [0,15]"; xmtfifosize8 "Transmit software FIFO size:"; xmtdatatype8 "Transmit FIFO data type:"; rcvfifosize8 "Receive software FIFO size:"
      mask help:
      | PMC521
      | Acromag
      | EIA/TIA-422B Send Receive Subsystem
      mask init:
      | brdslot = slot;
      | m_XR17D15x(1, 8);
      mask Help: helpview(fullfile(docroot, 'mapfiles', 'xpc.map'), 'Commtech_Subsystem')
      mask StyleString: popup(Board Setup|Basic Setup|FIFO Setup),popup(1|2|3|4|5|6|7|8),edit,edit,checkbox,edit,popup(921600|460800|230400|115200|57600|38400|19200|9600|4800|2400|1200|600|300|110),edit,popup(8x|16x (standard)),checkbox,popup(None|Even|Odd|Mark|Space),popup(5|6|7|8),popup(1|2),popup(1|quarter full (16)|half full (32)|almost full (56)),popup(RTS/CTS|none),popup(XON/XOFF|none),edit,edit,checkbox,edit,edit,popup(count+32 bit int|count+32 bit uint|count+16 bit int|count+16 bit uint|8 bit int null terminated|8 bit uint null terminated),edit,popup(921600|460800|230400|115200|57600|38400|19200|9600|4800|2400|1200|600|300|110),edit,popup(8x|16x (standard)),checkbox,popup(None|Even|Odd|Mark|Space),popup(5|6|7|8),popup(1|2),popup(1|quarter full (16)|half full (32)|almost full (56)),popup(RTS/CTS|none),popup(XON/XOFF|none),edit,edit,checkbox,edit,edit,popup(count+32 bit int|count+32 bit uint|count+16 bit int|count+16 bit uint|8 bit int null terminated|8 bit uint null terminated),edit,popup(921600|460800|230400|115200|57600|38400|19200|9600|4800|2400|1200|600|300|110),edit,popup(8x|16x (standard)),checkbox,popup(None|Even|Odd|Mark|Space),popup(5|6|7|8),popup(1|2),popup(1|quarter full (16)|half full (32)|almost full (56)),popup(RTS/CTS|none),popup(XON/XOFF|none),edit,edit,checkbox,edit,edit,popup(count+32 bit int|count+32 bit uint|count+16 bit int|count+16 bit uint|8 bit int null terminated|8 bit uint null terminated),edit,popup(921600|460800|230400|115200|57600|38400|19200|9600|4800|2400|1200|600|300|110),edit,popup(8x|16x (standard)),checkbox,popup(None|Even|Odd|Mark|Space),popup(5|6|7|8),popup(1|2),popup(1|quarter full (16)|half full (32)|almost full (56)),popup(RTS/CTS|none),popup(XON/XOFF|none),edit,edit,checkbox,edit,edit,popup(count+32 bit int|count+32 bit uint|count+16 bit int|count+16 bit uint|8 bit int null terminated|8 bit uint null terminated),edit,popup(921600|460800|230400|115200|57600|38400|19200|9600|4800|2400|1200|600|300|110),edit,popup(8x|16x (standard)),checkbox,popup(None|Even|Odd|Mark|Space),popup(5|6|7|8),popup(1|2),popup(1|quarter full (16)|half full (32)|almost full (56)),popup(RTS/CTS|none),popup(XON/XOFF|none),edit,edit,checkbox,edit,edit,popup(count+32 bit int|count+32 bit uint|count+16 bit int|count+16 bit uint|8 bit int null terminated|8 bit uint null terminated),edit,popup(921600|460800|230400|115200|57600|38400|19200|9600|4800|2400|1200|600|300|110),edit,popup(8x|16x (standard)),checkbox,popup(None|Even|Odd|Mark|Space),popup(5|6|7|8),popup(1|2),popup(1|quarter full (16)|half full (32)|almost full (56)),popup(RTS/CTS|none),popup(XON/XOFF|none),edit,edit,checkbox,edit,edit,popup(count+32 bit int|count+32 bit uint|count+16 bit int|count+16 bit uint|8 bit int null terminated|8 bit uint null terminated),edit,popup(921600|460800|230400|115200|57600|38400|19200|9600|4800|2400|1200|600|300|110),edit,popup(8x|16x (standard)),checkbox,popup(None|Even|Odd|Mark|Space),popup(5|6|7|8),popup(1|2),popup(1|quarter full (16)|half full (32)|almost full (56)),popup(RTS/CTS|none),popup(XON/XOFF|none),edit,edit,checkbox,edit,edit,popup(count+32 bit int|count+32 bit uint|count+16 bit int|count+16 bit uint|8 bit int null terminated|8 bit uint null terminated),edit,popup(921600|460800|230400|115200|57600|38400|19200|9600|4800|2400|1200|600|300|110),edit,popup(8x|16x (standard)),checkbox,popup(None|Even|Odd|Mark|Space),popup(5|6|7|8),popup(1|2),popup(1|quarter full (16)|half full (32)|almost full (56)),popup(RTS/CTS|none),popup(XON/XOFF|none),edit,edit,checkbox,edit,edit,popup(count+32 bit int|count+32 bit uint|count+16 bit int|count+16 bit uint|8 bit int null terminated|8 bit uint null terminated),edit
      mask CallbackString:
      | m_XR17D15x(2, 8);|m_XR17D15x(2, 8);|||m_XR17D15x(2, 8);
      | |||||||||||||||||||||||||||||||||||||||||||||||||||||||||||||||||||||||||||||||||||||||||||||||||||||||||||||||||||||||||||||||||||||||||
      mask Display:
      | disp('Acromag\nPMC521\nEIA-422B\nSend\nReceive');
      | port_label( 'input', 1, 'XMT1' );
      | port_label( 'input', 2, 'XMT2' );
      | port_label( 'input', 3, 'XMT3' );
      | port_label( 'input', 4, 'XMT4' );
      | port_label( 'input', 5, 'XMT5' );
      | port_label( 'input', 6, 'XMT6' );
      | port_label( 'input', 7, 'XMT7' );
      | port_label( 'input', 8, 'XMT8' );
      | 
      | port_label( 'output', 1, 'FIFO1' );
      | port_label( 'output', 2, 'FIFO2' );
      | port_label( 'output', 3, 'FIFO3' );
      | port_label( 'output', 4, 'FIFO4' );
      | port_label( 'output', 5, 'FIFO5' );
      | port_label( 'output', 6, 'FIFO6' );
      | port_label( 'output', 7, 'FIFO7' );
      | port_label( 'output', 8, 'FIFO8' );
